simulink model "sim_model"  (R2020b)
settings: Solver=VariableStepAuto  StartTime=0.0  StopTime=10.0  RelTol=1e-3
libraries: simulink_extras x1
settings Model: Creator=Admin  LastModifiedBy=Admin
settings SolverCC: AlgebraicLoopSolver=LineSearch

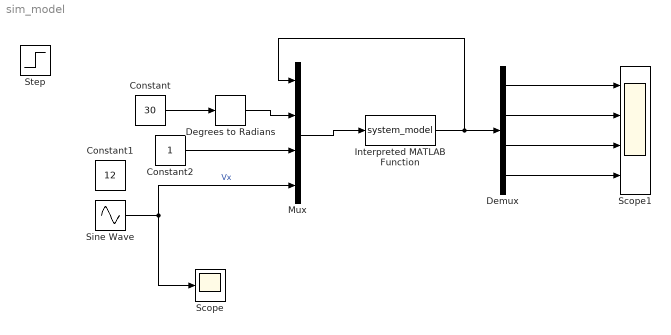
== system sim_model ==
  Constant : Constant  Value=30
  Constant1 : Constant  Value=12
  Constant2 : Constant
  Degrees to Radians : simulink_extras/Transformations/Degrees to Radians
  Demux : Demux
  Interpreted MATLAB Function : MATLABFcn  MATLABFcn=system_model  OutputDimensions=4
  Mux : Mux
  Scope : Scope
  Scope1 : Scope  NumInputPorts=4
  Sine Wave : Sin  SampleTime=0
  Step : Step  SampleTime=0
  wires:
  Mux/1 -> Interpreted MATLAB Function/1
  Interpreted MATLAB Function/1 -> Mux/1, Demux/1
  Sine Wave/1 -> Mux/4, Scope/1  "Vx"
  Demux/1 -> Scope1/1
  Demux/2 -> Scope1/2
  Demux/3 -> Scope1/3
  Demux/4 -> Scope1/4
  Degrees to Radians/1 -> Mux/2
  Constant/1 -> Degrees to Radians/1
  Constant2/1 -> Mux/3
